simulink model "DetailedReactormdl"  (R2020a)
settings: Solver=VariableStepAuto  StartTime=0.0  StopTime=10.0  RelTol=1e-3
settings Model: Creator=marce  LastModifiedBy=marce

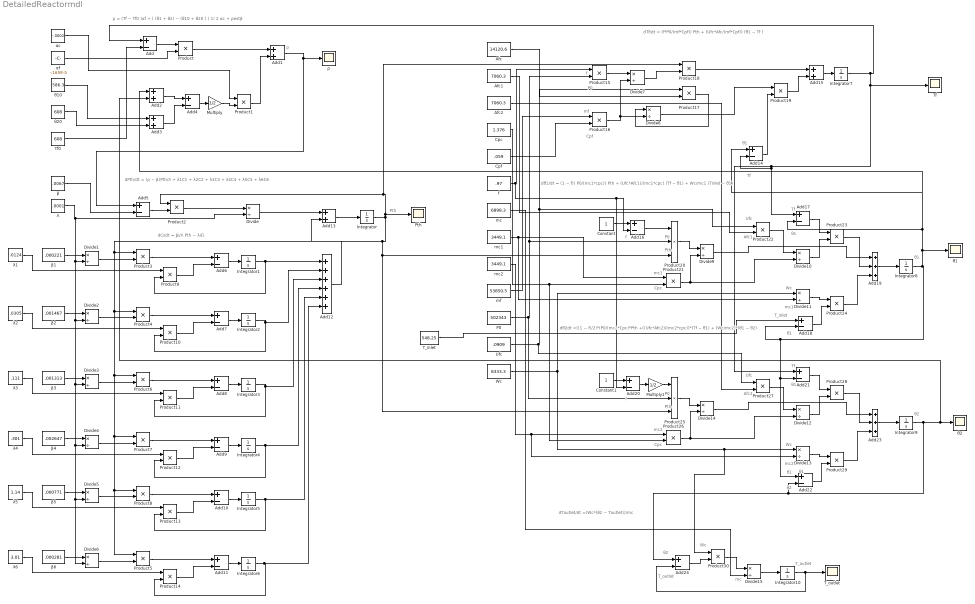
== system DetailedReactormdl ==
  note: T_outlet
  note: mc
  note: Wc
  note: T_outlet
  note: dToutlet/dt =(Wc*(θ2 − Toutlet))/mc
  note: dθ2dt =((1 − f)/2)*(P0/(mc2*Cpc)*Pth +((Ufc*Afc2)/(mc2*cpc))*(Tf − θ1) + (Wc/mc2)*(θ1 − θ2)
  note: dθ1/dt = (1 − f)( P0/(mc1*cpc)) Pth + (Ufc*Afc1)/(mc1*cpc) (Tf − θ1) + Wc/mc1 (Tinlet − θ1)
  note: T_inlet
  note: mc1
  note: Wc
  note: Tf
  note: Afc1
  note: Ufc
  note: Cpc
  note: mc1
  note: Pth
  note: P0
  note: f
  note: Cpf
  note: mf
  note: P0
  note: f
  note: θ1
  note: Tf
  note: dTf/dt = (f*P0/(mf*Cpf)) Pth + (Ufc*Afc/(mf*Cpf)) (θ1 − Tf )
  note: dCi/dt = βi/Λ Pth − λiCi
  note: Pth
  note: dPth/dt = (ρ − β)Pth/Λ + λ1C1 + λ2C2 + λ3C3 + λ4C4 + λ5C5 + λ6C6
  note: ρ
  note: ρ = (Tf − Tf0 )αf + ( (θ1 + θ2) − (θ10 + θ20 ) ) 1/ 2 αc + ρextβ
  note: θ1
  note: θ1
  note: θ1
  note: f
  note: mc2
  note: Pth
  note: Ufc
  note: Afc2
  note: θ2
  note: Tf
  note: mc2
  note: P0
  note: θ1
  note: θ1
  note: Cpc
  note: Wc
  note: θ1
  note: θ2
  note: θ2
  Add{,4..11,14,16..18,20..22,24} (17 alike) : Sum  Inputs=+-
  Add{1..3,13,15} (5 alike) : Sum
  Add12 : Sum  Inputs=++++++
  Add19 : Sum  Inputs=+++
  Add23 : Sum  Inputs=+++
  Afc : Constant  Value=14120.6
  Afc1 : Constant  Value=7060.3
  Afc2 : Constant  Value=7060.3
  Constant : Constant
  Constant1 : Constant
  Cpc : Constant  Value=1.376
  Cpf : Constant  Value=.059
  Divide{,1..15} (16 alike) : Product  Inputs=*/
  Integrator : Integrator  InitialCondition=.000001
  Integrator{1..10} (10 alike) : Integrator
  Multiply : Gain  Gain=1/2
  Multiply1 : Gain  Gain=1/2
  P0 : Constant  Value=502343
  Product{,1..19,21..24,26..30} (29 alike) : Product
  Product20 : Product  Inputs=3
  Product25 : Product  Inputs=3
  Pth : Scope
  T_inlet : Constant  Value=548.25
  T_outlet : Scope
  Tf : Scope
  Tf0 : Constant  Value=608
  Ufc : Constant  Value=.0909
  Wc : Constant  Value=8333.3
  f : Constant  Value=.97
  mc : Constant  Value=6898.3
  mc1 : Constant  Value=3449.1
  mc2 : Constant  Value=3449.1
  mf : Constant  Value=53850.5
  "Λ " : Constant  Value=.0001
  αc : Constant  Value=-.0002
  αf : Constant  Value=-.165E-5
  β : Constant  Value=.0067
  β1 : Constant  Value=.000221
  β2 : Constant  Value=.001467
  β3 : Constant  Value=.001313
  β4 : Constant  Value=.002647
  β5 : Constant  Value=.000771
  β6 : Constant  Value=.000281
  θ1 : Scope
  "θ10 " : Constant  Value=586.3
  θ2 : Scope
  θ20 : Constant  Value=608
  λ1 : Constant  Value=.0124
  λ2 : Constant  Value=.0305
  λ3 : Constant  Value=.111
  λ4 : Constant  Value=.301
  λ5 : Constant  Value=1.14
  λ6 : Constant  Value=3.01
  ρ : Scope
  wires:
  Tf0/1 -> Add/2
  Add/1 -> Product/1
  αf/1 -> Product/2
  Product/1 -> Add1/1
  "θ10 "/1 -> Add3/1
  θ20/1 -> Add3/2
  Add2/1 -> Add4/1
  Add3/1 -> Add4/2
  Add4/1 -> Multiply/1
  Multiply/1 -> Product1/2
  αc/1 -> Product1/1
  Product1/1 -> Add1/2
  Add1/1 -> Add5/1, ρ/1
  β/1 -> Add5/2
  Add5/1 -> Product2/2
  Integrator/1 -> Pth/1, Product18/1, Product2/1, Product25/3, Product20/3, Product5/1, Product8/1, Product7/1, Product6/1, Product4/1, Product3/1
  Product2/1 -> Divide/1
  "Λ "/1 -> Divide6/2, Divide5/2, Divide4/2, Divide3/2, Divide2/2, Divide1/2, Divide/2
  β1/1 -> Divide1/1
  β2/1 -> Divide2/1
  β3/1 -> Divide3/1
  β4/1 -> Divide4/1
  β5/1 -> Divide5/1
  β6/1 -> Divide6/1
  Divide1/1 -> Product3/2
  Divide2/1 -> Product4/2
  Divide3/1 -> Product6/2
  Divide4/1 -> Product7/2
  Divide5/1 -> Product8/2
  Divide6/1 -> Product5/2
  Add6/1 -> Integrator1/1
  Integrator1/1 -> Product9/2, Add12/1
  Product9/1 -> Add6/2
  Product3/1 -> Add6/1
  λ1/1 -> Product9/1
  λ2/1 -> Product10/1
  Add7/1 -> Integrator2/1
  Integrator2/1 -> Add12/2, Product10/2
  Product10/1 -> Add7/2
  Product4/1 -> Add7/1
  λ3/1 -> Product11/1
  Add8/1 -> Integrator3/1
  Integrator3/1 -> Add12/3, Product11/2
  Product11/1 -> Add8/2
  Product6/1 -> Add8/1
  λ4/1 -> Product12/1
  Add9/1 -> Integrator4/1
  Integrator4/1 -> Add12/4, Product12/2
  Product12/1 -> Add9/2
  Product7/1 -> Add9/1
  λ5/1 -> Product13/1
  Add10/1 -> Integrator5/1
  Integrator5/1 -> Add12/5, Product13/2
  Product13/1 -> Add10/2
  Product8/1 -> Add10/1
  λ6/1 -> Product14/1
  Add11/1 -> Integrator6/1
  Integrator6/1 -> Add12/6, Product14/2
  Product14/1 -> Add11/2
  Product5/1 -> Add11/1
  Add12/1 -> Add13/2
  Divide/1 -> Add13/1
  Add13/1 -> Integrator/1
  f/1 -> Add20/2, Add16/2, Product15/1
  P0/1 -> Product25/2, Product20/2, Product15/2
  Product15/1 -> Divide7/1
  Cpf/1 -> Product16/2
  mf/1 -> Product16/1
  Product16/1 -> Divide7/2, Divide8/2
  Afc/1 -> Product17/2
  Ufc/1 -> Product27/1, Product22/1, Product17/1
  Product17/1 -> Divide8/1
  Divide7/1 -> Product18/2
  Divide8/1 -> Product19/1
  Add14/1 -> Product19/2
  Product18/1 -> Add15/1
  Product19/1 -> Add15/2
  Add15/1 -> Integrator7/1
  Integrator7/1 -> Add/1, Tf/1, Add21/1, Add17/1, Add14/2
  Constant/1 -> Add16/1
  Add16/1 -> Product20/1
  Product20/1 -> Divide9/1
  Product21/1 -> Divide10/2, Divide9/2
  Product22/1 -> Divide10/1
  Add17/1 -> Product23/1
  Divide10/1 -> Product23/2
  Divide11/1 -> Product24/1
  Add18/1 -> Product24/2
  Divide9/1 -> Add19/1
  Product23/1 -> Add19/2
  Product24/1 -> Add19/3
  Add19/1 -> Integrator8/1
  Constant1/1 -> Add20/1
  Product27/1 -> Divide12/1
  Product29/1 -> Add23/3
  Divide14/1 -> Add23/1
  Add21/1 -> Product28/1
  Divide12/1 -> Product28/2
  Product28/1 -> Add23/2
  Add23/1 -> Integrator9/1
  Product25/1 -> Divide14/1
  Product26/1 -> Divide12/2, Divide14/2
  Divide13/1 -> Product29/1
  Add22/1 -> Product29/2
  Integrator8/1 -> θ1/1, Add2/1, Add14/1, Add17/2, Add18/2, Add22/1, Add21/2
  T_inlet/1 -> Add18/1
  Wc/1 -> Divide11/1, Product30/1, Divide13/1
  mc1/1 -> Divide11/2, Product21/1
  Cpc/1 -> Product26/2, Product21/2
  Afc1/1 -> Product22/2
  Add20/1 -> Multiply1/1
  Multiply1/1 -> Product25/1
  Integrator9/1 -> Add24/1, Add22/2, Add2/2, θ2/1
  mc2/1 -> Divide13/2, Product26/1
  Afc2/1 -> Product27/2
  Add24/1 -> Product30/2
  Product30/1 -> Divide15/1
  mc/1 -> Divide15/2
  Divide15/1 -> Integrator10/1
  Integrator10/1 -> Add24/2, T_outlet/1
